simulink model "ABS_V2"  (R2022a)
settings: Solver=VariableStepAuto  StartTime=0.0  StopTime=30  RelTol=1e-3
undefined symbols (not defined in the file): sigbuilder_block
settings Model: Creator=DELL  LastModifiedBy=DELL
settings ConfigComp: CovScope=ReferencedModels

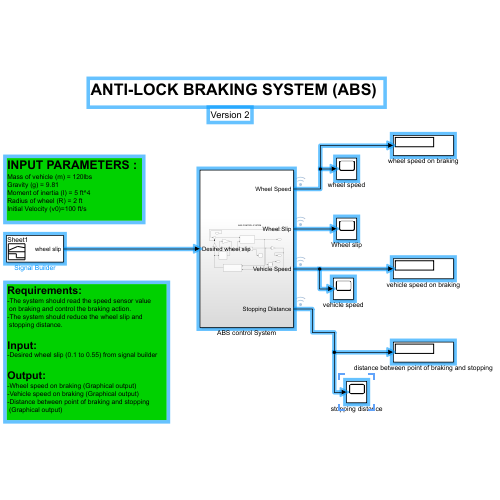
[thumbnail: Simulink's stored preview of the top-level diagram]
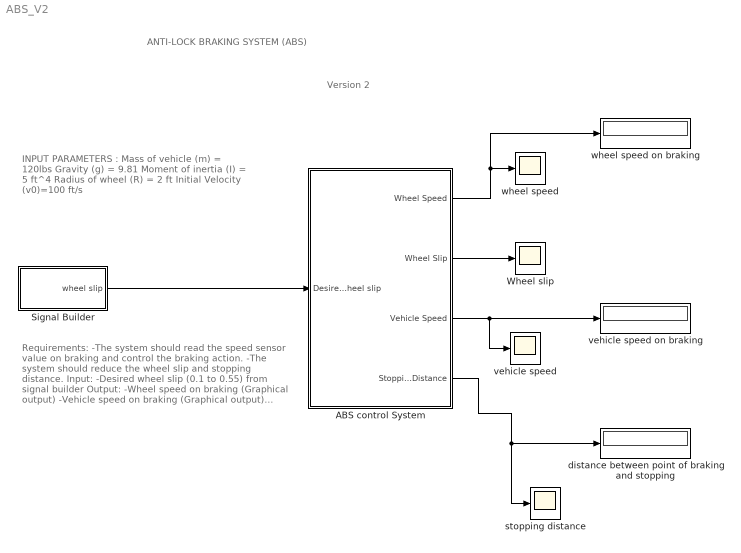
== system ABS_V2 ==
  note: INPUT PARAMETERS :
      | Mass of vehicle (m) = 120lbs
      | Gravity (g) = 9.81
      | Moment of inertia (I) = 5 ft^4
      | Radius of wheel (R) = 2 ft
      | Initial Velocity (v0)=100 ft/s
  note: Version 2
  note: ANTI-LOCK BRAKING SYSTEM (ABS)
  note: Requirements:
      | -The system should read the speed sensor value
      | on braking and control the braking action.
      | -The system should reduce the wheel slip and
      | stopping distance.
      |
      | Input:
      | -Desired wheel slip (0.1 to 0.55) from signal builder
      |
      | Output:
      | -Wheel speed on braking (Graphical output)
      | -Vehicle speed on braking (Graphical output)
      | -Distance between point of braking and stopping
      | (Graphical output)
  ABS control System : Subsystem
  Signal Builder : Subsystem  Tag=STV Subsys  LoadFcn=sigbuilder_block('load');  StartFcn=sigbuilder_block('start');  StopFcn=sigbuilder_block('stop');  ClipboardFcn=sigbuilder_block('clipboard');  mask(Sigbuilder block){tuvar=[0:10]}
      mask help: Simulink:masks:SigbuilderBlock_MD
      mask init:
      | if ~strcmp(get_param(bdroot(gcbh),'SimulationStatus'),'stopped') tuvar = sigbuilder_block('maskInit'); end
      settings: CopyFcn=sigbuilder_block('copy');  DeleteFcn=sigbuilder_block('delete');  ModelCloseFcn=sigbuilder_block('modelClose');  PreSaveFcn=sigbuilder_block('preSave');  PauseFcn=sigbuilder_block('pause');  ContinueFcn=sigbuilder_block('continue');  NameChangeFcn=sigbuilder_block('namechange');  OpenFcn=sigbuilder_block('open',[437.6 199.2 550.4 400 ]);  CloseFcn=sigbuilder_block('close');
      mask Display: plot(0, 0, 100, 100,[2, 2, 32, 32, 2], [68, 8, 8, 68, 68],[32, 2], [38, 38], [32, 19, 2],[53, 60, 44], [32, 17, 17, 2],[16, 16, 31, 31]);txt = getActiveGroup(gcbh);text(2, 100, txt,'verticalAlignment', 'top');
  Wheel slip : Scope
  distance between point of braking and stopping : Display
  stopping distance : Scope
  vehicle speed : Scope
  vehicle speed on braking : Display
  wheel speed : Scope
  wheel speed on braking : Display
  wires:
  ABS control System/3(Vehicle Speed) -> vehicle speed on braking/1, vehicle speed/1
  ABS control System/1(Wheel Speed) -> wheel speed/1, wheel speed on braking/1
  ABS control System/4(Stopping Distance) -> distance between point of braking and stopping/1, stopping distance/1
  Signal Builder/1(wheel slip) -> ABS control System/1(Desired wheel slip)
  ABS control System/2(Wheel Slip) -> Wheel slip/1

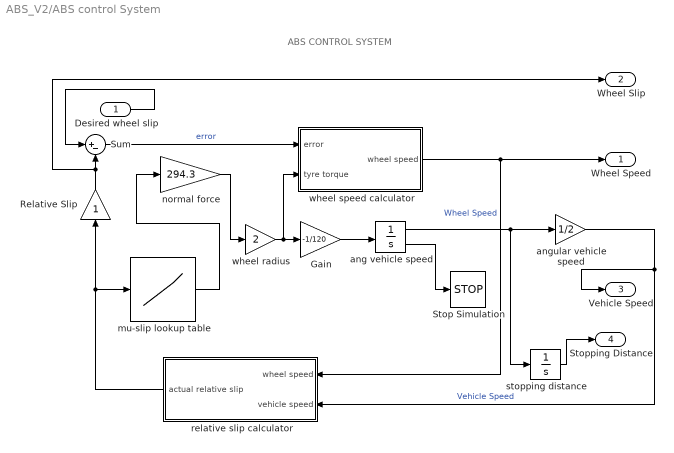
== system ABS_V2/ABS control System ==
  note: ABS CONTROL SYSTEM
  Desired wheel slip : Inport
  Gain : Gain  Gain=-1/120
  Relative Slip : Gain
  Stop Simulation : Stop
  Sum : Sum  Inputs=|+-
  ang vehicle speed : Integrator  InitialCondition=100  LimitOutput=on  UpperSaturationLimit=1000  LowerSaturationLimit=0  ShowSaturationPort=on
  angular vehicle speed : Gain  Gain=1/2
  mu-slip lookup table : Lookup_n-D  NumberOfTableDimensions=1  BreakpointsForDimension1=[0;0.05;0.1;0.15;0.2;0.25;0.3;0.35;0.4;0.45;0.5;0.55;0.6;0.65;0.7;0.75;0.8;0.85;0.9;0.95;1]  Table=[0;0.4;0.8;0.97;1;0.98;0.96;0.94;0.92;0.9;0.88;0.855;0.83;0.81;0.79;0.77;0.75;0.73;0.72;0.71;0.7]  InternalRulePriority=Speed  RndMeth=Simplest
  normal force : Gain  Gain=294.3
  relative slip calculator : Subsystem
  stopping distance : Integrator
  wheel radius : Gain  Gain=2
  wheel speed calculator : Subsystem
  Wheel Speed : Outport
  Wheel Slip : Outport  Port=2
  Vehicle Speed : Outport  Port=3
  Stopping Distance : Outport  Port=4
  wires:
  ang vehicle speed/1 -> angular vehicle speed/1, stopping distance/1
  relative slip calculator/1(actual relative slip) -> Relative Slip/1, mu-slip lookup table/1
  normal force/1 -> wheel radius/1
  wheel speed calculator/1(wheel speed) -> Wheel Speed/1, relative slip calculator/1(wheel speed)  "Wheel Speed"
  Sum/1 -> wheel speed calculator/1(error)  "error"
  angular vehicle speed/1 -> Vehicle Speed/1, relative slip calculator/2(vehicle speed)  "Vehicle Speed"
  Gain/1 -> ang vehicle speed/1
  wheel radius/1 -> Gain/1, wheel speed calculator/2(tyre torque)
  ang vehicle speed/2 -> Stop Simulation/1
  Relative Slip/1 -> Wheel Slip/1, Sum/2
  mu-slip lookup table/1 -> normal force/1
  stopping distance/1 -> Stopping Distance/1
  Desired wheel slip/1 -> Sum/1

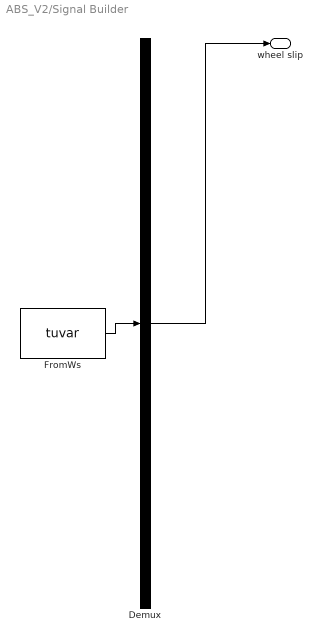
== system ABS_V2/Signal Builder ==
  Demux : Demux  Tag=STV Demux  Outputs=1
      settings: DisplayOption=none
  FromWs : FromWorkspace  Tag=STV FromWs  VariableName=tuvar
      SigBuilderData=|
      | common.afterFinalStr = 'Extrapolate'
      | common.sampleTime = 0
      | dataSet.timeRange = [1 10]
      | dataSet.name = 'Sheet1'
      | sbobj.Groups.Name = 'Sheet1'
      | sbobj.Groups.Signals.Name = 'wheel slip'
      | sbobj.Groups.Signals.XData = [1 2 3 4 5 6 7 8 9 10]
      | sbobj.Groups.Signals.YData = [0.1 0.15 0.2 0.25 0.3 0.35 0.4 0.45 0.5 0.55]
      | sbobj.Groups.TimeRange = [1 10]
  wheel slip : Outport  Tag=STV Outport
  wires:
  Demux/1 -> wheel slip/1
  FromWs/1 -> Demux/1

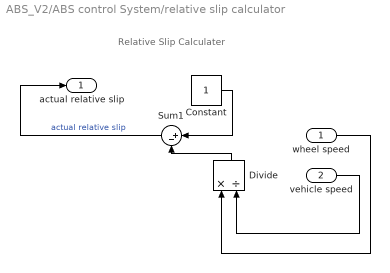
== system ABS_V2/ABS control System/relative slip calculator ==
  note: Relative Slip Calculater
  wheel speed : Inport
  vehicle speed : Inport  Port=2
  Constant : Constant
  Divide : Product  Inputs=*/
  Sum1 : Sum  Inputs=|+-
  actual relative slip : Outport
  wires:
  Divide/1 -> Sum1/2
  vehicle speed/1 -> Divide/2
  wheel speed/1 -> Divide/1
  Sum1/1 -> actual relative slip/1  "actual relative slip"
  Constant/1 -> Sum1/1

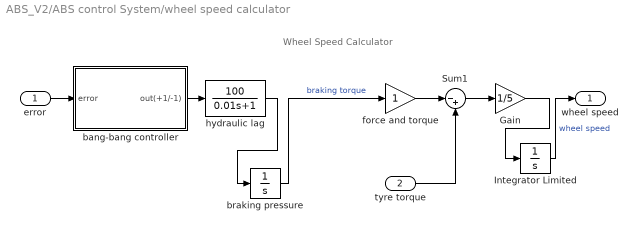
== system ABS_V2/ABS control System/wheel speed calculator ==
  note: Wheel Speed Calculator
  error : Inport
  tyre torque : Inport  Port=2
  Gain : Gain  Gain=1/5
  Integrator Limited : Integrator  InitialCondition=100/2  LimitOutput=on  UpperSaturationLimit=1000  LowerSaturationLimit=0
  Sum1 : Sum  Inputs=|-+
  bang-bang controller : Subsystem
  braking pressure : Integrator  LimitOutput=on  UpperSaturationLimit=1000  LowerSaturationLimit=0
  force and torque : Gain
  hydraulic lag : TransferFcn  Numerator=[100]  Denominator=[0.01 1]
  wheel speed : Outport
  wires:
  bang-bang controller/1(out(+1/-1)) -> hydraulic lag/1
  hydraulic lag/1 -> braking pressure/1
  Integrator Limited/1 -> wheel speed/1  "wheel speed"
  Sum1/1 -> Gain/1
  error/1 -> bang-bang controller/1(error)
  braking pressure/1 -> force and torque/1  "braking torque"
  Gain/1 -> Integrator Limited/1
  tyre torque/1 -> Sum1/2
  force and torque/1 -> Sum1/1

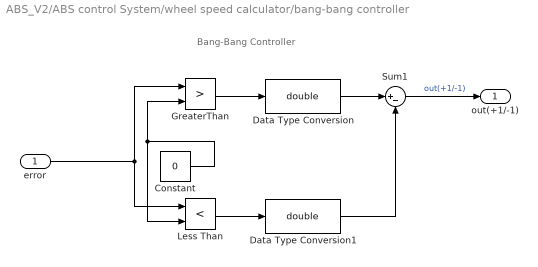
== system ABS_V2/ABS control System/wheel speed calculator/bang-bang controller ==
  note: Bang-Bang Controller
  error : Inport
  Constant : Constant  Value=0
  Data Type Conversion : DataTypeConversion  OutDataTypeStr=double  SaturateOnIntegerOverflow=off
  Data Type Conversion1 : DataTypeConversion  OutDataTypeStr=double  SaturateOnIntegerOverflow=off
  GreaterThan : RelationalOperator  Operator=>  OutDataTypeStr=boolean  RndMeth=Simplest  InputSameDT=off
  Less Than : RelationalOperator  Operator=<  OutDataTypeStr=boolean  RndMeth=Simplest  InputSameDT=off
  Sum1 : Sum  Inputs=|+-
  out(+1/-1) : Outport
  wires:
  Constant/1 -> GreaterThan/2, Less Than/2
  Data Type Conversion/1 -> Sum1/1
  GreaterThan/1 -> Data Type Conversion/1
  Less Than/1 -> Data Type Conversion1/1
  error/1 -> GreaterThan/1, Less Than/1
  Data Type Conversion1/1 -> Sum1/2
  Sum1/1 -> out(+1/-1)/1  "out(+1/-1)"
